simulink model "Pendule"  (R2021a)
settings: Solver=VariableStepAuto  StartTime=0.0  StopTime=10.0  RelTol=1e-3
libraries: simulink x1
settings Model: Creator=lmeissne  LastModifiedBy=lmeissne

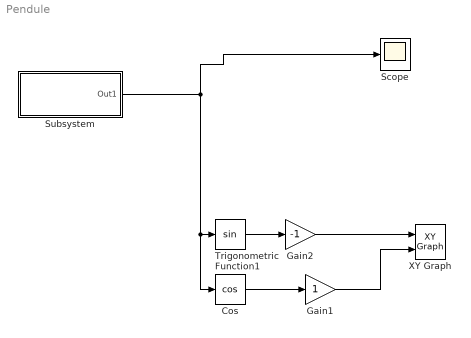
== system Pendule ==
  Cos : Trigonometry  Operator=cos
  Gain1 : Gain
  Gain2 : Gain  Gain=-1
  Scope : Scope
  Subsystem : Subsystem
  Trigonometric Function1 : Trigonometry
  XY Graph : simulink/Sinks/XY Graph  xmin=-1  xmax=1  ymin=-1  ymax=1  st=-1
  wires:
  Cos/1 -> Gain1/1
  Trigonometric Function1/1 -> Gain2/1
  Gain1/1 -> XY Graph/2
  Gain2/1 -> XY Graph/1
  Subsystem/1(Out1) -> Cos/1, Trigonometric Function1/1, Scope/1

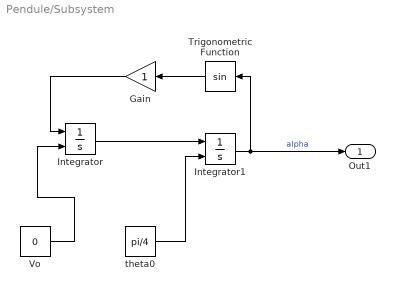
== system Pendule/Subsystem ==
  Gain : Gain
  Integrator : Integrator  InitialConditionSource=external
  Integrator1 : Integrator  InitialConditionSource=external
  Trigonometric Function : Trigonometry
  Vo : Constant  Value=0
  theta0 : Constant  Value=pi/4
  Out1 : Outport
  wires:
  Trigonometric Function/1 -> Gain/1
  Integrator1/1 -> Out1/1, Trigonometric Function/1  "alpha"
  theta0/1 -> Integrator1/2
  Gain/1 -> Integrator/1
  Integrator/1 -> Integrator1/1
  Vo/1 -> Integrator/2
